simulink model "flightControl"  (R2015b)
settings: Solver=FixedStepDiscrete  StartTime=0.0  StopTime=inf  FixedStep=1/1000  RelTol=1e-3
libraries: simulink x1, embdlinuxlib x1, quadLibrary x1
settings Model: SimulationMode=external  ExtModeEnableFloating=off  ExtModeTrigDuration=100  Creator=Nik Descher  LastModifiedBy=Nik Descher
settings DataIOCC: LimitDataPoints=off
settings OptimizationCC: OptimizeModelRefInitCode=on  LifeSpan=1
settings HardwareCC: ProdBitPerPointer=32  ProdLargestAtomicInteger=Long  ProdLargestAtomicFloat=Double  ProdWordSize=32  ProdHWDeviceType=ARM Compatible->ARM Cortex
settings RTWCC: SystemTargetFile=realtime.tlc  GenerateMakefile=off  TemplateMakefile=realtime.tmf  Description=Run on Target Hardware  RTWVerbose=off
settings STFCustomTargetCC: TargetLibSuffix=.a  GenerateSampleERTMain=on  ConcurrentExecutionCompliant=off  GeneratePreprocessorConditionals=Use local settings  ERTCustomFileBanners=on  SupportNonInlinedSFcns=off  SupportVariableSizeSignals=on  MATLABClassNameForMDSCustomization=Simulink.SoftwareTarget.ERTCustomization  CPPClassGenCompliant=off  GRTInterface=off  SystemTargetFile=realtime.tlc
settings ERTTargetCC: GenerateSampleERTMain=on  ParMdlRefBuildCompliant=off  CompOptLevelCompliant=off  ConcurrentExecutionCompliant=off  CombineOutputUpdateFcns=off  ERTFirstTimeCompliant=off  SupportContinuousTime=on  SupportVariableSizeSignals=on  ModelStepFunctionPrototypeControlCompliant=off  CPPClassGenCompliant=off  UseToolchainInfoCompliant=off  ExtModeMexArgs='192.168.1.248' 0 17724  ERTSrcFileBannerTemplate=realtime_code_template.cgt  ERTHdrFileBannerTemplate=realtime_code_template.cgt  ERTDataSrcFileTemplate=realtime_code_template.cgt  ERTDataHdrFileTemplate=realtime_code_template.cgt  ERTCustomFileTemplate=realtime_file_process.tlc

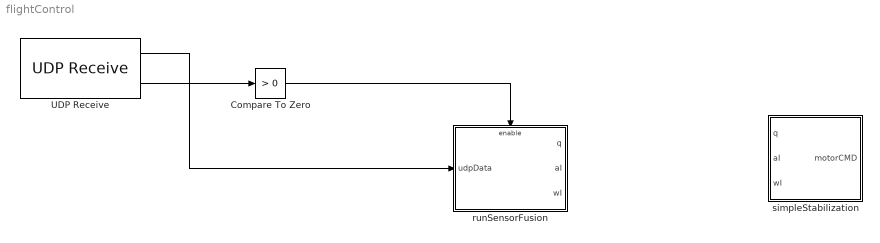
== system flightControl ==
  Compare To Zero : simulink/Logic and Bit Operations/Compare To Zero  relop=>  OutDataTypeStr=boolean
  UDP Receive : embdlinuxlib/UDP Receive  localURL='0.0.0.0'  localPort=25000  remoteURL='0.0.0.0'  remotePort=-1  recvBufferSize=8192  signalDatatype=single  dims=31  isVarSize=off  showBlockingTime=off  blockingTime=0  sampletime=1/1000  blockPlatform=Raspberry Pi
  runSensorFusion : Subsystem  TreatAsAtomicUnit=on
  simpleStabilization : Subsystem
  wires:
  UDP Receive/1 -> runSensorFusion/1(udpData)
  UDP Receive/2 -> Compare To Zero/1
  Compare To Zero/1 -> runSensorFusion/Enable

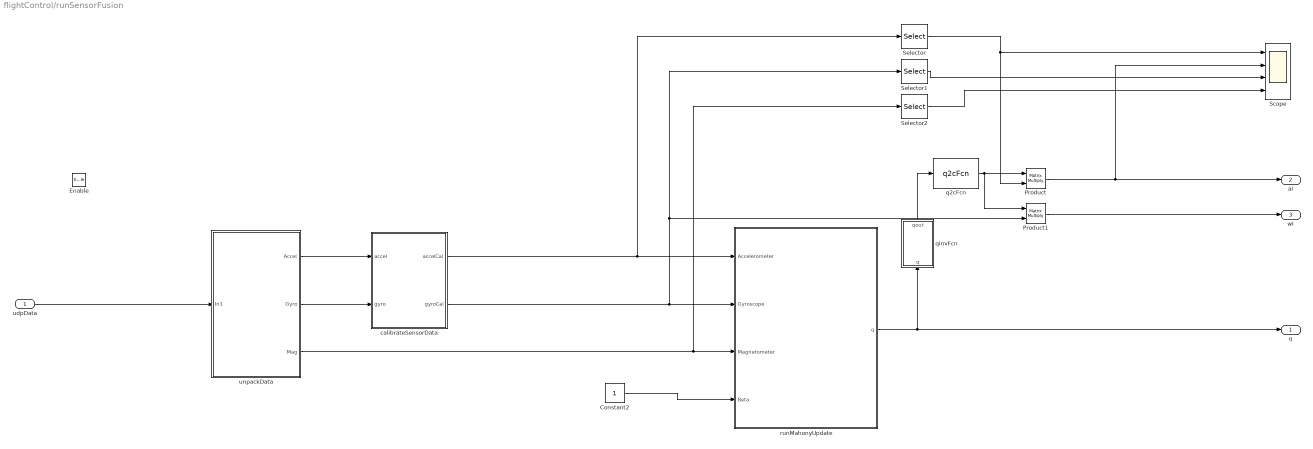
== system flightControl/runSensorFusion ==
  udpData : Inport
  Enable : EnablePort
  Constant2 : Constant  OutDataTypeStr=single
  Product : Product  Multiplication=Matrix(*)
  Product1 : Product  Multiplication=Matrix(*)
  Scope : Scope  NumInputPorts=4
  Selector : Selector  NumberOfDimensions=2  InputPortWidth=3  IndexOptions=Index vector (dialog),Index vector (dialog)  Indices=[1 2 3],4  OutputSizes=1,1
  Selector1 : Selector  NumberOfDimensions=2  InputPortWidth=3  IndexOptions=Index vector (dialog),Index vector (dialog)  Indices=[1 2 3],4  OutputSizes=1,1
  Selector2 : Selector  NumberOfDimensions=2  InputPortWidth=3  IndexOptions=Index vector (dialog),Index vector (dialog)  Indices=[1 2 3],2  OutputSizes=1,1
  calibrateSensorData : Subsystem
  q2cFcn : quadLibrary/q2cFcn
  qinvFcn : MATLAB Function  TreatAsAtomicUnit=on
  runMahonyUpdate : MATLAB Function  TreatAsAtomicUnit=on
  unpackData : Subsystem
  q : Outport
  aI : Outport  Port=2
  wI : Outport  Port=3
  wires:
  Constant2/1 -> runMahonyUpdate/4(Beta)
  runMahonyUpdate/1(q) -> q/1, qinvFcn/1(q)
  unpackData/3(Mag) -> runMahonyUpdate/3(Magnetometer), Selector2/1
  udpData/1 -> unpackData/1(In1)
  unpackData/1(Accel) -> calibrateSensorData/1(accel)
  unpackData/2(Gyro) -> calibrateSensorData/2(gyro)
  calibrateSensorData/1(accelCal) -> Selector/1, runMahonyUpdate/1(Accelerometer)
  calibrateSensorData/2(gyroCal) -> runMahonyUpdate/2(Gyroscope), Selector1/1, Product1/2
  q2cFcn/1 -> Product1/1, Product/1
  Product/1 -> aI/1, Scope/2
  Selector/1 -> Product/2, Scope/1
  Selector1/1 -> Scope/3
  Selector2/1 -> Scope/4
  qinvFcn/1(qout) -> q2cFcn/1
  Product1/1 -> wI/1

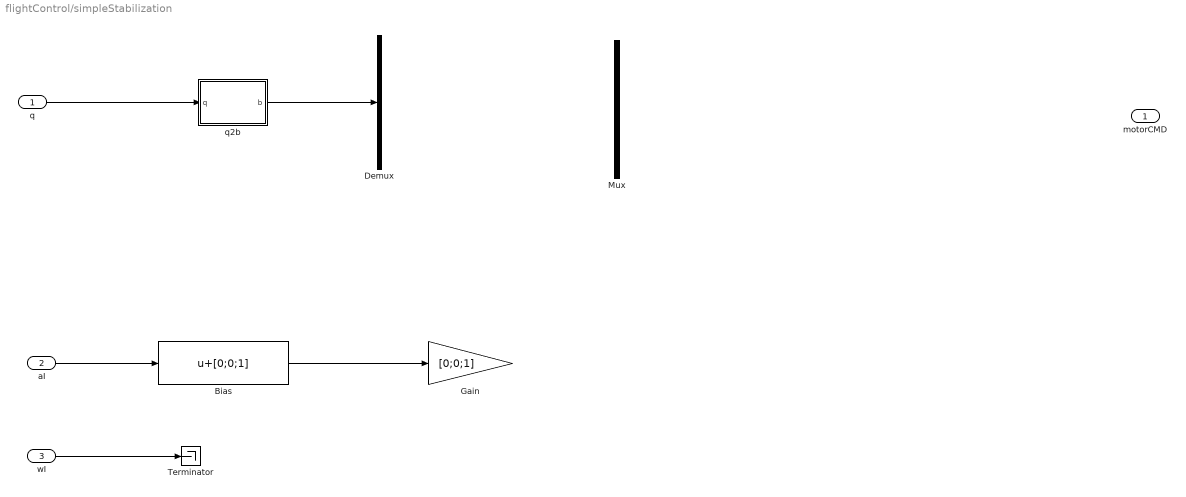
== system flightControl/simpleStabilization ==
  q : Inport
  aI : Inport  Port=2
  wI : Inport  Port=3
  Bias : Bias  Bias=[0;0;1]
  Demux : Demux  Outputs=3
  Gain : Gain  Gain=[0;0;1]
  Mux : Mux
  Terminator : Terminator
  q2b : MATLAB Function  TreatAsAtomicUnit=on
  motorCMD : Outport
  wires:
  aI/1 -> Bias/1
  Bias/1 -> Gain/1
  wI/1 -> Terminator/1
  q/1 -> q2b/1(q)
  q2b/1(b) -> Demux/1

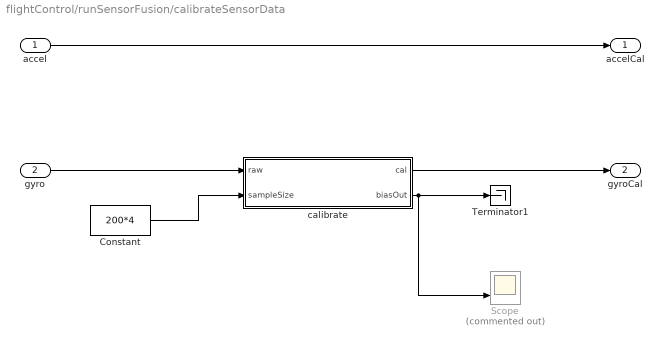
== system flightControl/runSensorFusion/calibrateSensorData ==
  accel : Inport
  gyro : Inport  Port=2
  Constant : Constant  Value=200*4  OutDataTypeStr=single
  Scope : Scope  Commented=on  NumInputPorts=2
  Terminator1 : Terminator
  calibrate : MATLAB Function  TreatAsAtomicUnit=on
  accelCal : Outport
  gyroCal : Outport  Port=2
  wires:
  accel/1 -> accelCal/1
  calibrate/1(cal) -> gyroCal/1
  calibrate/2(biasOut) -> Scope/2, Terminator1/1
  gyro/1 -> calibrate/1(raw)
  Constant/1 -> calibrate/2(sampleSize)

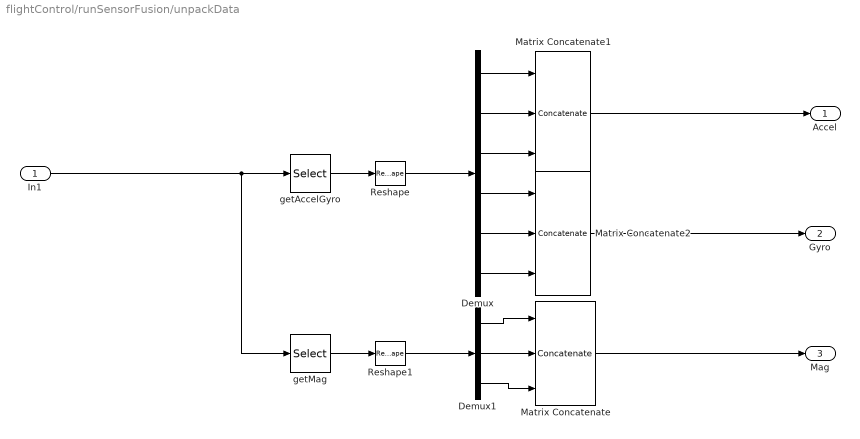
== system flightControl/runSensorFusion/unpackData ==
  In1 : Inport
  Demux : Demux  Outputs=6
  Demux1 : Demux  Outputs=3
  Matrix Concatenate : Concatenate  NumInputs=3  Mode=Multidimensional array
  Matrix Concatenate1 : Concatenate  NumInputs=3  Mode=Multidimensional array
  Matrix Concatenate2 : Concatenate  NumInputs=3  Mode=Multidimensional array
  Reshape : Reshape
  Reshape1 : Reshape
  getAccelGyro : Selector  InputPortWidth=31  IndexOptions=Index vector (dialog)  Indices=1:24  OutputSizes=1
  getMag : Selector  InputPortWidth=31  IndexOptions=Index vector (dialog)  Indices=25:30  OutputSizes=1
  Accel : Outport
  Gyro : Outport  Port=2
  Mag : Outport  Port=3
  wires:
  In1/1 -> getMag/1, getAccelGyro/1
  getMag/1 -> Reshape1/1
  Reshape1/1 -> Demux1/1
  Demux1/2 -> Matrix Concatenate/2
  Demux1/1 -> Matrix Concatenate/1
  Demux1/3 -> Matrix Concatenate/3
  Demux/2 -> Matrix Concatenate1/2
  Demux/3 -> Matrix Concatenate1/3
  Demux/1 -> Matrix Concatenate1/1
  Demux/4 -> Matrix Concatenate2/1
  Demux/5 -> Matrix Concatenate2/2
  Reshape/1 -> Demux/1
  getAccelGyro/1 -> Reshape/1
  Demux/6 -> Matrix Concatenate2/3
  Matrix Concatenate2/1 -> Gyro/1
  Matrix Concatenate/1 -> Mag/1
  Matrix Concatenate1/1 -> Accel/1

== matlab function flightControl/simpleStabilization/q2b ==
  data: q input; b output
function b=q2b(q)
%#codegen
% Q2B converts a quaternion (q) to a Bortz vector (b).
%
%  usage: b=q2b(q)
%
%     q = qnb
%
%     where q(1)   = scalar part
%           q(2-4) = vector part
%
b=zeros(3,1);
%
if (q(1) < 0.0)
  q=-q;
end
%
qs=q(1);
qv=[q(2);q(3);q(4)];
%
theta=single(2)*acos(qs);
%
if (theta > 1.0e-20) 
  st=sin(theta/2);
  ux=qv(1)/st;
  uy=qv(2)/st;
  uz=qv(3)/st;
  b=theta*[ux;uy;uz];
end

== matlab function flightControl/runSensorFusion/runMahonyUpdate ==
  data: Accelerometer input single size=[3 4]; q output single size=[ 4 1]; Gyroscope input single size=[3 4]; Magnetometer input single size=[3 2]; Beta input single size=1
function q  = runMadwickUpdates(Accelerometer,Gyroscope,Magnetometer,Beta)
persistent qLocal
if isempty(qLocal)
    qLocal=single([1 0 0 0]');
end
qIn=qLocal;



magInterp=interp1([1 4],Magnetometer',[1 2 3 4],'linear')';

for i=1:4
    
    q  = runMadwickUpdate(qIn,Accelerometer(:,i),Gyroscope(:,i),magInterp(:,i),Beta);
    qIn = q;
    
end

qLocal=q;

function q  = runMadwickUpdate(qIn,Accelerometer,Gyroscope,Magnetometer,Beta)
q=qIn;
SamplePeriod=single(5/1000);

% Normalise accelerometer measurement
if ~all(abs(Accelerometer)<.0001);
    Accelerometer = Accelerometer / norm(Accelerometer);	% normalise magnitude
end
% Normalise magnetometer measurement
if ~all(abs(Magnetometer)<.0001)
    Magnetometer = Magnetometer / norm(Magnetometer);	% normalise magnitude
end
% Reference direction of Earth's magnetic feild
h = quaternProd(q, quaternProd([0 Magnetometer'], quaternConj(q)));
b = [0 norm([h(2) h(3)]) 0 h(4)];
% Gradient decent algorithm corrective step
F = [2*(q(2)*q(4) - q(1)*q(3)) - Accelerometer(1)
    2*(q(1)*q(2) + q(3)*q(4)) - Accelerometer(2)
    2*(0.5 - q(2)^2 - q(3)^2) - Accelerometer(3)
    2*b(2)*(0.5 - q(3)^2 - q(4)^2) + 2*b(4)*(q(2)*q(4) - q(1)*q(3)) - Magnetometer(1)
    2*b(2)*(q(2)*q(3) - q(1)*q(4)) + 2*b(4)*(q(1)*q(2) + q(3)*q(4)) - Magnetometer(2)
    2*b(2)*(q(1)*q(3) + q(2)*q(4)) + 2*b(4)*(0.5 - q(2)^2 - q(3)^2) - Magnetometer(3)];
J = [-2*q(3),                 	2*q(4),                    -2*q(1),                         2*q(2)
    2*q(2),                 	2*q(1),                    	2*q(4),                         2*q(3)
    0,                         -4*q(2),                    -4*q(3),                         0
    -2*b(4)*q(3),               2*b(4)*q(4),               -4*b(2)*q(3)-2*b(4)*q(1),       -4*b(2)*q(4)+2*b(4)*q(2)
    -2*b(2)*q(4)+2*b(4)*q(2),	2*b(2)*q(3)+2*b(4)*q(1),	2*b(2)*q(2)+2*b(4)*q(4),       -2*b(2)*q(1)+2*b(4)*q(3)
    2*b(2)*q(3),                2*b(2)*q(4)-4*b(4)*q(2),	2*b(2)*q(1)-4*b(4)*q(3),        2*b(2)*q(2)];
step = (J'*F);
step = step / norm(step);	% normalise step magnitude

% Compute rate of change of quaternion
qDot = 0.5 * quaternProd(q, [0; Gyroscope(1); Gyroscope(2); Gyroscope(3)]) - Beta * step;

% Integrate to yield quaternion
q = q + qDot * SamplePeriod;
q = q / norm(q); % normalise quaternion


function ab = quaternProd(a, b)
    ab=zeros(4,1);
%QUATERNPROD Calculates the quaternion product
%
%   ab = quaternProd(a, b)
%
%   Calculates the quaternion product of quaternion a and b.
%
%   For more information see:
%   http://www.x-io.co.uk/node/8#quaternions
%
%	Date          Author          Notes
%	27/09/2011    SOH Madgwick    Initial release

    ab(1) = a(1).*b(1)-a(2).*b(2)-a(3).*b(3)-a(4).*b(4);
    ab(2) = a(1).*b(2)+a(2).*b(1)+a(3).*b(4)-a(4).*b(3);
    ab(3) = a(1).*b(3)-a(2).*b(4)+a(3).*b(1)+a(4).*b(2);
    ab(4) = a(1).*b(4)+a(2).*b(3)-a(3).*b(2)+a(4).*b(1);

function qConj = quaternConj(q)
%QUATERN2ROTMAT Converts a quaternion to its conjugate
%
%   qConj = quaternConj(q)
%
%   Converts a quaternion to its conjugate.
%
%   For more information see:
%   http://www.x-io.co.uk/node/8#quaternions
%
%	Date          Author          Notes
%	27/09/2011    SOH Madgwick    Initial release

    qConj = [q(1); -q(2); -q(3); -q(4)];

== matlab function flightControl/runSensorFusion/calibrateSensorData/calibrate ==
  data: raw input single size=[3 4]; cal output single size=[3 4]; biasOut output; sampleSize input
function [cal,biasOut] = calFcn(raw,sampleSize)
%#codegen

persistent bias count
if isempty(count)
    count=uint32(1);
    bias=single(zeros(3,1));
end

if count>=sampleSize
    cal=raw-[bias bias bias bias];
else
    cal=single(zeros(3,4));
    for i=1:4
        bias=bias+single((1/sampleSize)).*raw(:,i);
        count=count+1;    
    end
end
biasOut=bias;

== matlab function flightControl/runSensorFusion/qinvFcn ==
  data: q input single size=[4 1]; qout output single size=[4 1]
function qout=qinv(q)
%#codegen

%
qout=[q(1);
      -q(2:4)];
